simulink model "RI_RL_ISZM"  (R2013b)
settings: Solver=ode45  StartTime=0.0  StopTime=10e-3  MaxStep=(1e-6)/2  RelTol=1e-3
libraries: RI_MK x3
settings Model: Creator=Szalay  LastModifiedBy=Szalay

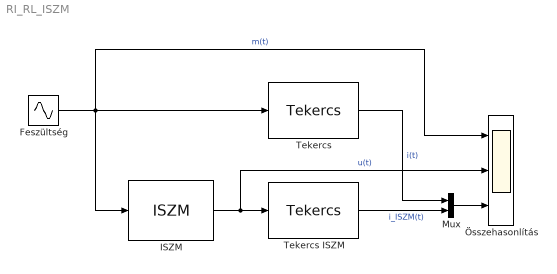
== system RI_RL_ISZM ==
  Feszültség : Sin  Amplitude=6  Frequency=2*pi*100  SampleTime=0
  ISZM : RI_MK/ISZM  U_T=12  f_ISZM=25000  T_S=0.25e-6
  Mux : Mux  Inputs=2
  Tekercs : RI_MK/Tekercs  R=1  L=1e-3  i_0=0
  Tekercs ISZM : RI_MK/Tekercs  R=1  L=1e-3  i_0=0
  Összehasonlítás : Scope  NumInputPorts=3
      settings: ShowLegends=on  TimeRange=0.01  YMin=-6~-15~-6  YMax=6~15~6
  wires:
  ISZM/1 -> Összehasonlítás/2, Tekercs ISZM/1  "u(t)"
  Feszültség/1 -> ISZM/1, Összehasonlítás/1, Tekercs/1  "m(t)"
  Mux/1 -> Összehasonlítás/3
  Tekercs/1 -> Mux/1  "i(t)"
  Tekercs ISZM/1 -> Mux/2  "i_ISZM(t)"
